simulink model "Receiver"  (R2023a)
settings: Solver=FixedStepAuto  StartTime=0.0  StopTime=10.0  RelTol=1e-3
undefined symbols (not defined in the file): FINAL_recerver_1, latitude, longitude
libraries: androidcommunicationlib x4, androidaudiovideolib x2, androiduilib x2
settings Model: Creator=VENKAT  LastModifiedBy=mohit
settings OptimizationCC: EnhancedBackFolding=on  PassReuseOutputArgsAs=Individual arguments  ZeroExternalMemoryAtStartup=off  ZeroInternalMemoryAtStartup=off  MaxStackSize=64  OptimizeBlockOrder=speed  DifferentSizesBufferReuse=on  OptimizationCustomize=off  EfficientTunableParamExpr=on
settings DebuggingCC: ParameterTunabilityLossMsg=error
settings HardwareCC: ProdBitPerPointer=32  ProdBitPerSizeT=32  ProdBitPerPtrDiffT=32  ProdLargestAtomicInteger=Long  ProdLargestAtomicFloat=Double  ProdWordSize=32  ProdHWDeviceType=ARM Compatible->ARM Cortex  UseEmbeddedCoderFeatures=off  UseSimulinkCoderFeatures=off
settings SFSimCC: MATLABDynamicMemAlloc=off
settings RTWCC: Description=Embedded Coder  SystemTargetFile=ert.tlc  HardwareBoard=Android Device  TLCOptions="-aInlineSetEventsForThisBaseRateFcn=TLC_FALSE -aSuppressMultiTaskScheduler=TLC_FALSE  -aRateBasedStepFcn=0"  TemplateMakefile=ert_default_tmf  RTWVerbose=off  Toolchain=Android SDK/NDK Tools
settings CodeAppCC: ForceParamTrailComments=on  IgnoreCustomStorageClasses=off  OperatorAnnotations=on  SimulinkDataObjDesc=on  SFDataObjDesc=on  InsertBlockDesc=on
settings ERTTargetCC: SupportNonInlinedSFcns=on

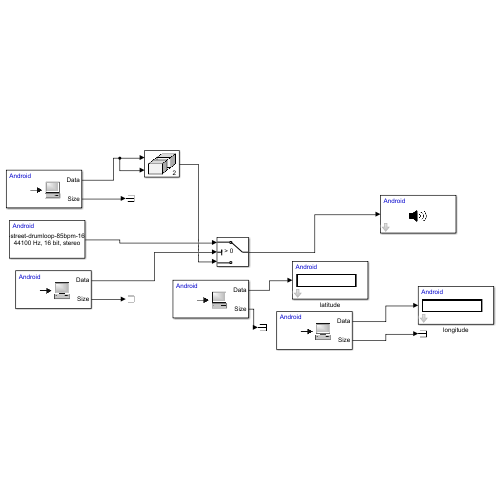
[thumbnail: Simulink's stored preview of the top-level diagram]
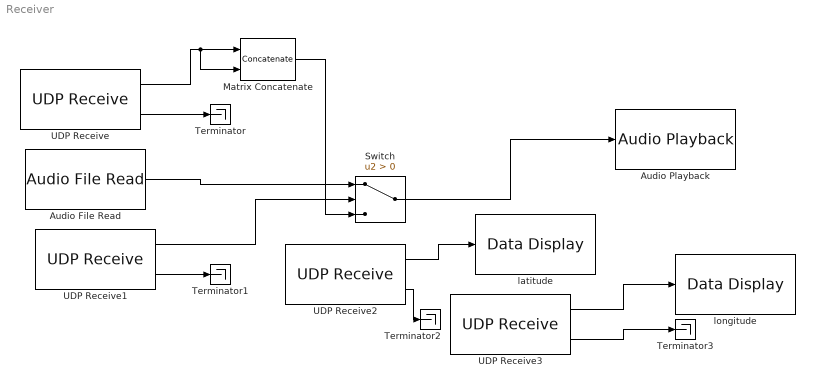
== system Receiver ==
  Audio File Read : androidaudiovideolib/Audio File Read  FileName=C:\Users\mohit\OneDrive\Desktop\acad\ssrp\sunflower-street-drumloop-85bpm-163900.mp3  FrameSize=441
  Audio Playback : androidaudiovideolib/Audio Playback  SampleFreq=44100  AudioSamplingFreq=44100  SampleTime=0.1  DeviceStr=0  QueueDuration=0  BlockPlatform=Android
  Matrix Concatenate : Concatenate  Mode=Multidimensional array  ConcatenateDimension=2
  Switch : Switch  Criteria=u2 > Threshold  OutDataTypeStr=int16  SaturateOnIntegerOverflow=off  InputSameDT=off
  Terminator{,1..3} (4 alike) : Terminator
  UDP Receive : androidcommunicationlib/UDP Receive  localURL='0.0.0.0'  localPort=25000  remoteURL='0.0.0.0'  remotePort=-1  recvBufferSize=8192  signalDatatype=int16  dims=441  isVarSize=off  showBlockingTime=off  blockingTime=0  sampletime=0.01  blockPlatform=Android
  UDP Receive1 : androidcommunicationlib/UDP Receive  localURL='0.0.0.0'  localPort=35000  remoteURL='0.0.0.0'  remotePort=-1  recvBufferSize=8192  signalDatatype=int16  dims=1  isVarSize=off  showBlockingTime=off  blockingTime=0  sampletime=0.01  blockPlatform=Android
  UDP Receive2 : androidcommunicationlib/UDP Receive  localURL='0.0.0.0'  localPort=30000  remoteURL='0.0.0.0'  remotePort=-1  recvBufferSize=8192  signalDatatype=double  dims=1  isVarSize=off  showBlockingTime=off  blockingTime=0  sampletime=0.01  blockPlatform=Android
  UDP Receive3 : androidcommunicationlib/UDP Receive  localURL='0.0.0.0'  localPort=40000  remoteURL='0.0.0.0'  remotePort=-1  recvBufferSize=8192  signalDatatype=double  dims=1  isVarSize=off  showBlockingTime=off  blockingTime=0  sampletime=0.01  blockPlatform=Android
  latitude : androiduilib/Data Display  DataDisplayId=FINAL_recerver_1/latitude  Format=Float  Precision=6  SimulateUsing=Code generation  blockPlatform=Android
  longitude : androiduilib/Data Display  DataDisplayId=FINAL_recerver_1/longitude  Format=Float  Precision=6  SimulateUsing=Code generation  blockPlatform=Android
  wires:
  UDP Receive1/1 -> Switch/2
  UDP Receive/1 -> Matrix Concatenate/2, Matrix Concatenate/1
  Matrix Concatenate/1 -> Switch/3
  Audio File Read/1 -> Switch/1
  Switch/1 -> Audio Playback/1
  UDP Receive1/2 -> Terminator1/1
  UDP Receive/2 -> Terminator/1
  UDP Receive2/2 -> Terminator2/1
  UDP Receive3/2 -> Terminator3/1
  UDP Receive2/1 -> latitude/1
  UDP Receive3/1 -> longitude/1
